simulink model "control"  (R2022b)
settings: Solver=VariableStepAuto  StartTime=0.0  StopTime=10.0  RelTol=1e-3
values from neighbouring files (symbols this model uses):
  k = 0.035    [date_indrumator.m]    (also in proiect.m)
  k11 = k2^2 + 4*(k - k3)*k1    (= 0.08909684)    [date_indrumator.m]    (also in proiect.m = 0.08885985)
  k12 = 8*(k-k3)    (= 0.2848)    [date_indrumator.m]    (also in proiect.m)
  k13 = 2*(k-k3)    (= 0.0712)    [date_indrumator.m]    (also in proiect.m)
  k2 = -0.015    [date_indrumator.m]    (also in proiect.m = -0.0015)
  keta = 8*(10^-5)    (= 8e-05)    [date_indrumator.m]    (also in proiect.m)
libraries: slpidlib x1
settings Model: Creator=Ruxandra  LastModifiedBy=Ruxandra

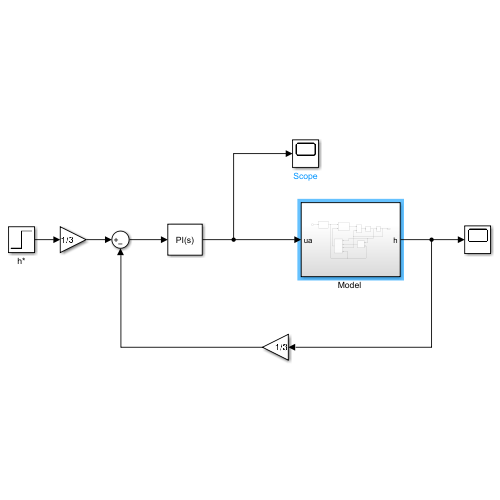
[thumbnail: Simulink's stored preview of the top-level diagram]
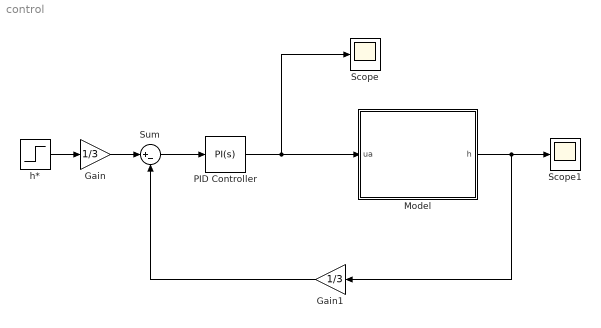
== system control ==
  Gain : Gain  Gain=1/3
  Gain1 : Gain  Gain=1/3
  "Model " : Subsystem
  PID Controller : slpidlib/PID Controller  Controller=PI  Form=Parallel  TimeDomain=Continuous-time  UseExternalTs=off  SampleTime=-1  IntegratorMethod=Forward Euler  FilterMethod=Forward Euler  ControllerParametersSource=internal  P=2.395  I=160  UseKiTs=off  D=0  N=100  UseFilter=on  TunerSelectOption=Transfer Function Based (PID Tuner App)  InitialConditionSource=internal  InitialConditionForIntegrator=0  InitialConditionForFilter=0  DifferentiatorICPrevScaledInput=0  ExternalReset=none  TrackingMode=off  Kt=1  LimitOutput=off  SatLimitsSource=internal  UpperSaturationLimit=inf  LowerSaturationLimit=-inf  LinearizeAsGain=on  AntiWindupMode=none  Kb=1  LimitIntegrator=off  UpperIntegratorSaturationLimit=inf  LowerIntegratorSaturationLimit=-inf  POutMin=[]  POutMax=[]  IOutMin=[]  IOutMax=[]  DOutMin=[]  DOutMax=[]  NOutMin=[]  NOutMax=[]  SumOutMin=[]  SumOutMax=[]  SaturationOutMin=[]  SaturationOutMax=[]  PParamMin=[]  PParamMax=[]  IParamMin=[]  IParamMax=[]  DParamMin=[]  DParamMax=[]  NParamMin=[]  NParamMax=[]  KbParamMin=[]  KbParamMax=[]  KtParamMin=[]  KtParamMax=[]  KbOutMin=[]  KbOutMax=[]  KtOutMin=[]  KtOutMax=[]  IntegratorOutMin=[]  IntegratorOutMax=[]  FilterOutMin=[]  FilterOutMax=[]  SumI1OutMin=[]  SumI1OutMax=[]  SumI2OutMin=[]  SumI2OutMax=[]  SumI3OutMin=[]  SumI3OutMax=[]  SumI4OutMin=[]  SumI4OutMax=[]  SumDOutMin=[]  SumDOutMax=[]  DifferentiatorOutMin=[]  DifferentiatorOutMax=[]  FilterDiffOutCoefMin=[]  FilterDiffOutCoefMax=[]  ReciprocalOutMin=[]  ReciprocalOutMax=[]  SumDenOutMin=[]  SumDenOutMax=[]  SumNumOutMin=[]  SumNumOutMax=[]  DivideOutMin=[]  DivideOutMax=[]  UdiffTsProdOutMin=[]  UdiffTsProdOutMax=[]  NTsProdOutMin=[]  NTsProdOutMax=[]  UintegralTsProdOutMin=[]  UintegralTsProdOutMax=[]  UngainTsProdOutMin=[]  UngainTsProdOutMax=[]  ClampingZeroOutDataTypeStr=Inherit: Inherit via back propagation  ClampingZeroOutMin=[]  ClampingZeroOutMax=[]  FilterDenConstantOutDataTypeStr=Inherit: Inherit via back propagation  FilterDenConstantOutMin=[]  FilterDenConstantOutMax=[]  PCopyOutDataTypeStr=Inherit: Inherit via back propagation  PCopyOutMin=[]  PCopyOutMax=[]  NCopyOutDataTypeStr=Inherit: Inherit via back propagation  NCopyOutMin=[]  NCopyOutMax=[]  IntegratorContinuousStateAttributes=''  IntegratorStateMustResolveToSignalObject=off  IntegratorRTWStateStorageClass=Auto  FilterContinuousStateAttributes=''  FilterStateMustResolveToSignalObject=off  FilterRTWStateStorageClass=Auto  ParallelPVariant=InternalParameters  IdealPVariant=Disabled  IVariant=InternalParameters  DVariant=Disabled  IntegratorVariant=Continuous  SatVariant=Disabled  AWVariant=Passthrough  PCopyVariant=Disabled  TRVariant=Disabled  FdbkBlocksVariant=Forward  IdealPFdbkVariant=Disabled  SatFdbkVariant=Disabled  DerivativeFilterVariant=Disabled  NVariant=Disabled  NCopyVariant=Disabled_SignalSpec  FilterICVariant=Disabled  IntegratorICVariant=InternalICs  ExternalResetVariant=Disabled  TRSumVariant=Passthrough  SumFdbkVariant=Disabled  SumVariant=Sum_PI  TsampFilterVariant=InternalTs  TsampNgainVariant=Passthrough  TsampIntegralVariant=Passthrough  ExternalSaturationOutDataTypeStr=Inherit: Same as second input
  Scope : Scope
  Scope1 : Scope
  Sum : Sum  Inputs=|+-
  h* : Step  SampleTime=0
  wires:
  h*/1 -> Gain/1
  Gain/1 -> Sum/1
  Sum/1 -> PID Controller/1
  PID Controller/1 -> Scope/1, "Model "/1(ua)
  "Model "/1(h) -> Gain1/1, Scope1/1
  Gain1/1 -> Sum/2

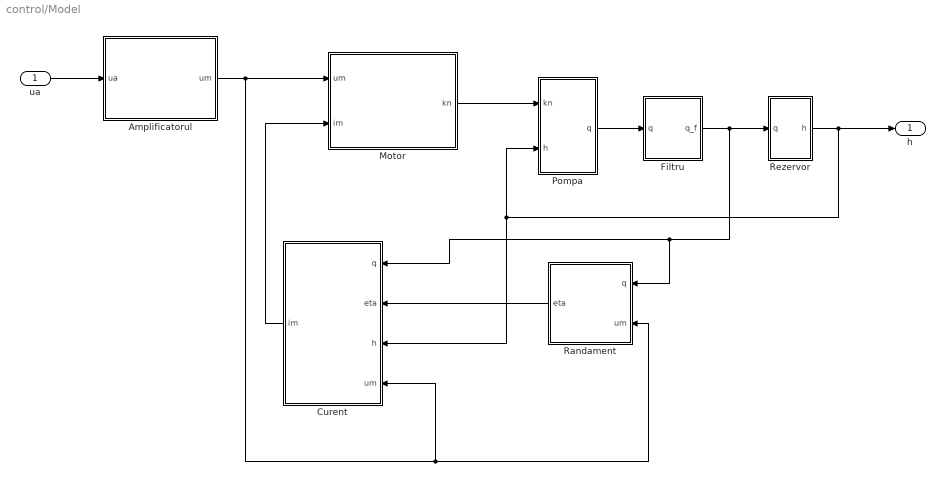
== system control/Model  ==
  ua : Inport
  Amplificatorul : Subsystem
  Curent : Subsystem
  Filtru : Subsystem
  Motor : Subsystem
  Pompa : Subsystem
  Randament : Subsystem
  Rezervor : Subsystem
  h : Outport
  wires:
  Amplificatorul/1(um) -> Motor/1(um), Curent/4(um), Randament/2(um)
  Rezervor/1(h) -> h/1, Pompa/2(h), Curent/3(h)
  Motor/1("kn ") -> Pompa/1(kn)
  ua/1 -> Amplificatorul/1(ua)
  Randament/1(eta) -> Curent/2(eta)
  Curent/1(im) -> Motor/2(im)
  Filtru/1(q_f) -> Rezervor/1(q), Curent/1(q), Randament/1(q)
  Pompa/1(q) -> Filtru/1(q)

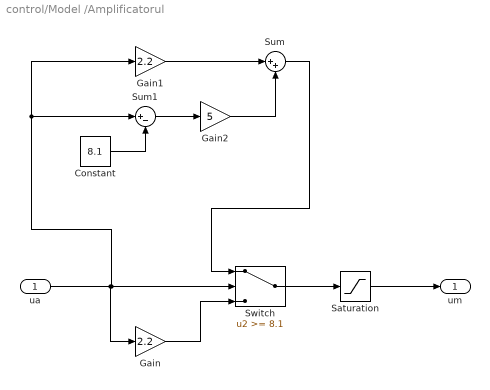
== system control/Model /Amplificatorul ==
  ua : Inport
  Constant : Constant  Value=8.1
  Gain : Gain  Gain=2.2
  Gain1 : Gain  Gain=2.2
  Gain2 : Gain  Gain=5
  Saturation : Saturate  UpperLimit=22  LowerLimit=0
  Sum : Sum  Inputs=|++
  Sum1 : Sum  Inputs=|+-
  Switch : Switch  Threshold=8.1  RndMeth=Nearest  SaturateOnIntegerOverflow=off  InputSameDT=off
  um : Outport
  wires:
  Gain1/1 -> Sum/1
  ua/1 -> Sum1/1, Gain1/1, Switch/2, Gain/1
  Saturation/1 -> um/1
  Gain/1 -> Switch/3
  Gain2/1 -> Sum/2
  Sum1/1 -> Gain2/1
  Sum/1 -> Switch/1
  Switch/1 -> Saturation/1
  Constant/1 -> Sum1/2

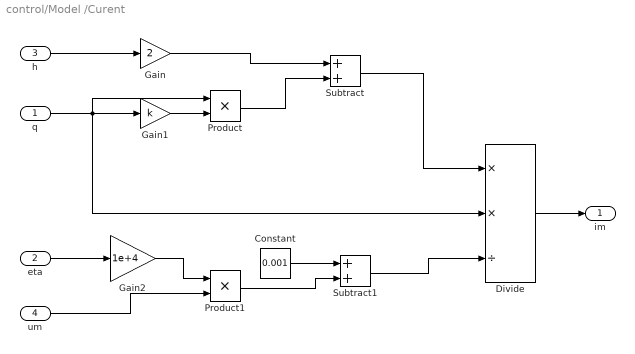
== system control/Model /Curent ==
  q : Inport
  eta : Inport  Port=2
  h : Inport  Port=3
  um : Inport  Port=4
  Constant : Constant  Value=0.001
  Divide : Product  Inputs=**/
  Gain : Gain  Gain=2
  Gain1 : Gain  Gain=k
  Gain2 : Gain  Gain=1e+4
  Product : Product
  Product1 : Product
  Subtract : Sum
  Subtract1 : Sum
  im : Outport
  wires:
  Product/1 -> Subtract/2
  h/1 -> Gain/1
  Gain/1 -> Subtract/1
  Subtract1/1 -> Divide/3
  Gain2/1 -> Product1/1
  Constant/1 -> Subtract1/1
  Subtract/1 -> Divide/1
  Gain1/1 -> Product/2
  eta/1 -> Gain2/1
  Product1/1 -> Subtract1/2
  q/1 -> Divide/2, Gain1/1, Product/1
  um/1 -> Product1/2
  Divide/1 -> im/1

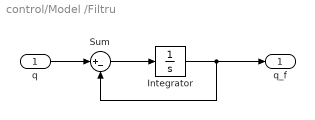
== system control/Model /Filtru ==
  q : Inport
  Integrator : Integrator
  Sum : Sum  Inputs=|+-
  q_f : Outport
  wires:
  q/1 -> Sum/1
  Integrator/1 -> q_f/1, Sum/2
  Sum/1 -> Integrator/1

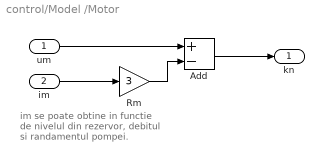
== system control/Model /Motor ==
  note: im se poate obtine in functie de nivelul din rezervor, debitul si randamentul pompei.
  um : Inport
  im : Inport  Port=2
  Add : Sum  Inputs=+-
  Rm : Gain  Gain=3
  "kn " : Outport
  wires:
  im/1 -> Rm/1
  um/1 -> Add/1
  Rm/1 -> Add/2
  Add/1 -> "kn "/1

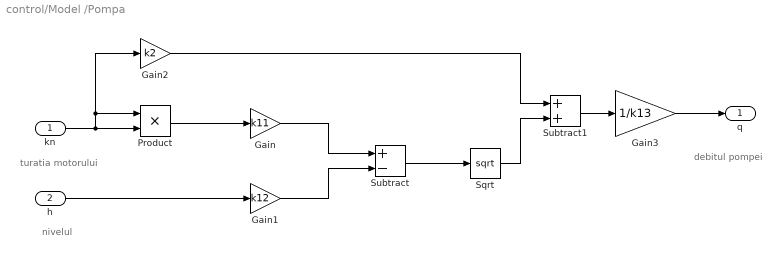
== system control/Model /Pompa ==
  note: debitul pompei
  note: nivelul
  note: turatia motorului
  kn : Inport
  h : Inport  Port=2
  Gain : Gain  Gain=k11
  Gain1 : Gain  Gain=k12
  Gain2 : Gain  Gain=k2
  Gain3 : Gain  Gain=1/k13
  Product : Product
  Sqrt : Sqrt
  Subtract : Sum  Inputs=+-
  Subtract1 : Sum
  q : Outport
  wires:
  Sqrt/1 -> Subtract1/2
  Gain1/1 -> Subtract/2
  h/1 -> Gain1/1
  Gain2/1 -> Subtract1/1
  kn/1 -> Product/1, Gain2/1, Product/2
  Subtract/1 -> Sqrt/1
  Subtract1/1 -> Gain3/1
  Gain/1 -> Subtract/1
  Gain3/1 -> q/1
  Product/1 -> Gain/1

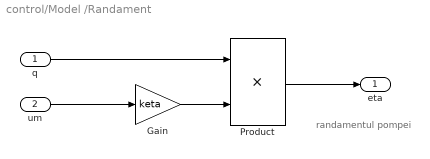
== system control/Model /Randament ==
  note: randamentul pompei
  q : Inport
  um : Inport  Port=2
  Gain : Gain  Gain=keta
  Product : Product
  eta : Outport
  wires:
  um/1 -> Gain/1
  Product/1 -> eta/1
  q/1 -> Product/1
  Gain/1 -> Product/2

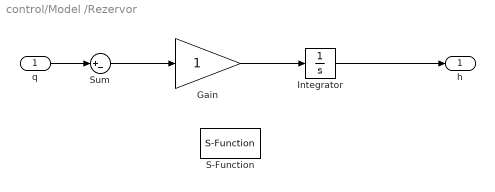
== system control/Model /Rezervor ==
  q : Inport
  Gain : Gain
  Integrator : Integrator
  S-Function : S-Function  SFunctionDeploymentMode=off  EnableBusSupport=off
  Sum : Sum  Inputs=|+-
  h : Outport
  wires:
  Integrator/1 -> h/1
  q/1 -> Sum/1
  Gain/1 -> Integrator/1
  Sum/1 -> Gain/1
